simulink model "pv_mpp"  (R2023b)
settings: Solver=ode23tb  StartTime=0.0  StopTime=inf  FixedStep=0.001  MaxStep=1e-4  RelTol=1e-4
libraries: spsSeriesRLCBranchLib x4, spsCurrentMeasurementLib x1, spsDiodeLib x1, spsIGBTDiodeLib x1, spsPVArrayLib x1, spsPWMGeneratorDCDCLib x1, spsVoltageMeasurementLib x1, sps_lib x1
settings Model: Creator=SAUMYA  LastModifiedBy=SAUMYA

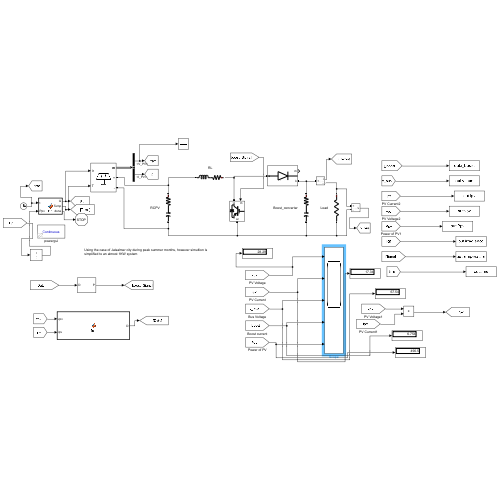
[thumbnail: Simulink's stored preview of the top-level diagram]
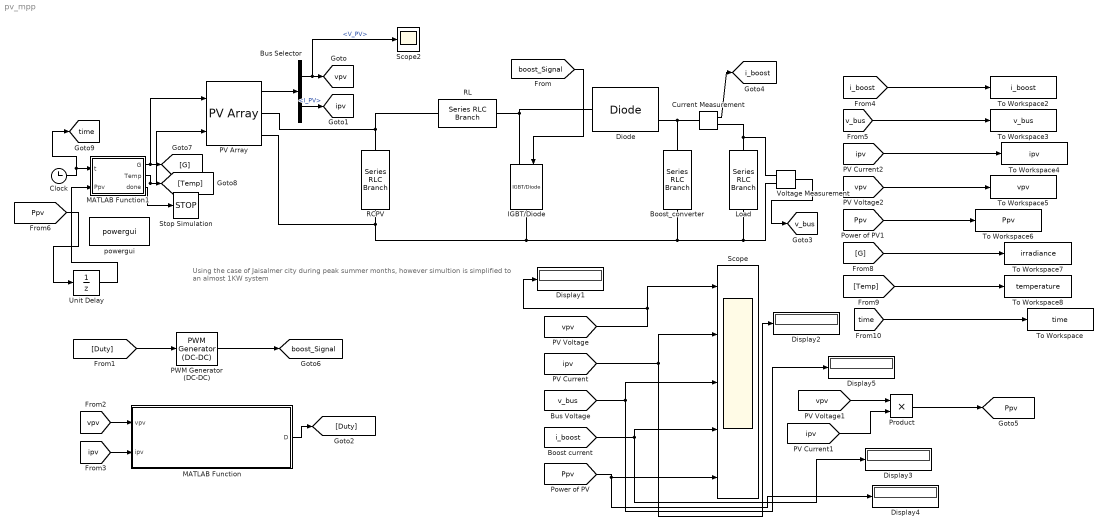
== system pv_mpp ==
  note: Using the case of Jaisalmer city during peak summer months, however simultion is simplified to an almost 1KW system
  Boost_converter : spsSeriesRLCBranchLib/Series RLC Branch  LConnTagsString=__new0  RConnTagsString=__new0  BranchType=RC  Resistance=1e-4  Inductance=1e-3  SetiL0=off  InitialCurrent=0  Capacitance=3300e-6  Setx0=on  InitialVoltage=0  Measurements=None
  Bus Selector : BusSelector  OutputSignals=V_PV,I_PV
  Clock : Clock
  Current Measurement : spsCurrentMeasurementLib/Current Measurement  PhasorSimulation=off  OutputType=Complex  PSBequivalent=0
  Diode : spsDiodeLib/Diode  Ron=0.001  Lon=0  Vf=0.8  IC=0  UseSnubber=0  Rs=inf  Cs=250e-9  Measurements=on
  Display{1..5} (5 alike) : Display
  IGBT/Diode : spsIGBTDiodeLib/IGBT//Diode  Ron=1e-3  Rs=1e5  Cs=inf  Measurements=off
  Load : spsSeriesRLCBranchLib/Series RLC Branch  LConnTagsString=__new0  RConnTagsString=__new0  BranchType=R  Resistance=10  Inductance=1e-3  SetiL0=off  InitialCurrent=0  Capacitance=3300e-6  Setx0=on  InitialVoltage=0  Measurements=None
  MATLAB Function : MATLAB Function  TreatAsAtomicUnit=on
  MATLAB Function1 : MATLAB Function  TreatAsAtomicUnit=on
  PV Array : spsPVArrayLib/PV Array  Npar=5  Nser=1  PlotType=array @ 1000 W/m2 & specified temperatures  S_vec="[ 1000  500  100 ]"  Temp_C_vec=[ 15 25 35 45 55 ]  ModuleName=Changzhou Almaden SEBP60S-220  PlotWhenSelected=off  Pm=219.876  Ncell=60  Voc=36.06  Isc=7.95  Vm=30.12  Im=7.3  beta_Voc_pc=-0.3624  alpha_Isc_pc=0.054805  beta_Voc=-0.13068  alpha_Isc=0.004357  IL=7.9642  I0=2.8692e-10  nI=0.97455  Rsh=106.1817  Rs=0.18964  RobustModel=off  RobustCellTemperature=313.3991  BAL=on  Tc=1e-6  Tfilter=5e-5
  PWM Generator (DC-DC) : spsPWMGeneratorDCDCLib/PWM Generator (DC-DC)  Fsw=5000  Ts=10e-6
  Product : Product
  RCPV : spsSeriesRLCBranchLib/Series RLC Branch  LConnTagsString=__new0  RConnTagsString=__new0  BranchType=RC  Resistance=1e-4  Inductance=1e-3  SetiL0=off  InitialCurrent=0  Capacitance=100e-6  Setx0=on  InitialVoltage=0  Measurements=None
  RL : spsSeriesRLCBranchLib/Series RLC Branch  LConnTagsString=__new0  RConnTagsString=__new0  BranchType=RL  Resistance=0.1  Inductance=5e-3  SetiL0=off  InitialCurrent=0  Capacitance=1e-3  Setx0=on  InitialVoltage=0  Measurements=None
  Scope : Scope  NumInputPorts=5
  Scope2 : Scope
  Stop Simulation : Stop
  To Workspace : ToWorkspace  VariableName=time  SampleTime=-1
  To Workspace2 : ToWorkspace  VariableName=i_boost  SampleTime=-1
  To Workspace3 : ToWorkspace  VariableName=v_bus  SampleTime=-1
  To Workspace4 : ToWorkspace  VariableName=ipv  SampleTime=-1
  To Workspace5 : ToWorkspace  VariableName=vpv  SampleTime=-1
  To Workspace6 : ToWorkspace  VariableName=Ppv  SampleTime=-1
  To Workspace7 : ToWorkspace  VariableName=irradiance  SampleTime=-1
  To Workspace8 : ToWorkspace  VariableName=temperature  SampleTime=-1
  Unit Delay : UnitDelay  SampleTime=-1  HasFrameUpgradeWarning=on
  Voltage Measurement : spsVoltageMeasurementLib/Voltage Measurement  PhasorSimulation=off  OutputType=Complex  PSBequivalent=0
  powergui : sps_lib/powergui  Priority=1  SimulationMode=Continuous  SampleTime=0.001  frequency=60  Iterations=50  frequencyindice=0  Pbase=100e6  ErrMax=1e-4  UnitsV=kV  UnitsW=MW  buscounter=0  FunctionMessages=off  echomessages=off  EnableUseOfTLC=off  CurrentSourceSwitches=off  DisableSnubberDevices=off  DisableRonSwitches=off  DisableVfSwitches=off  DisplayEquations=off  AutomaticDiscreteSolvers=off  SolverType=Tustin/Backward Euler (TBE)  Interpol=off  ExternalGateDelay=off  methode=off  Ts=100  x0status=blocks  SPID=on  SwTol=0  HookPort=off  NonlinearTolerance=1e-4  nMaxIteration=100  ContinueOnMaxIteration=off  RestoreLinks=warning  ResistiveCurrentMeasurement=off  Frange=[0:2:500]  Ylog=off  Xlog=on  ShowGrid=off  save=off  variable=ZData  structure=0  ZoomFFT=off  StartTime=0.0  cycles=1  DisplayStyle=1  fundamental=60  FreqAxis=off  MaxFrequency=1000  frequencyindicesteady=1  RmsSteady=1  display=off
  tag scope: Ppv=global, boost_Signal=global, i_boost=global, ipv=global, time=global, v_bus=global, vpv=global
  wires:
  Clock/1 -> [time], MATLAB Function1/1(t)
  MATLAB Function1/1(G) -> PV Array/1, [G]
  PWM Generator (DC-DC)/1 -> [boost_Signal]
  Current Measurement/1 -> [i_boost]
  [ipv] -> MATLAB Function/2(ipv)
  [vpv] -> Display1/1, Scope/1
  MATLAB Function1/2(Temp) -> PV Array/2, [Temp]
  [ipv] -> Product/2
  Bus Selector/1 -> Scope2/1, [vpv]  "<V_PV>"
  [v_bus] -> Display5/1, Scope/3
  [Duty] -> PWM Generator (DC-DC)/1
  Product/1 -> [Ppv]
  [boost_Signal] -> IGBT/Diode/1
  [i_boost] -> Display3/1, Scope/4
  [Ppv] -> Display4/1, Scope/5
  PV Array/1 -> Bus Selector/1
  MATLAB Function/1(D) -> [Duty]
  [vpv] -> MATLAB Function/1(vpv)
  [ipv] -> Display2/1, Scope/2
  [vpv] -> Product/1
  Voltage Measurement/1 -> [v_bus]
  Bus Selector/2 -> [ipv]  "<I_PV>"
  [i_boost] -> To Workspace2/1
  [v_bus] -> To Workspace3/1
  [ipv] -> To Workspace4/1
  [vpv] -> To Workspace5/1
  [Ppv] -> To Workspace6/1
  [G] -> To Workspace7/1
  [Temp] -> To Workspace8/1
  [time] -> To Workspace/1
  [Ppv] -> Unit Delay/1
  Unit Delay/1 -> MATLAB Function1/2(Ppv)
  MATLAB Function1/3(done) -> Stop Simulation/1
  connections:
  RCPV/LConn1 -- RL/RConn1 -- PV Array/RConn1
  RCPV/RConn1 -- Boost_converter/RConn1 -- Load/RConn1 -- Voltage Measurement/LConn2 -- IGBT/Diode/RConn1 -- PV Array/RConn2
  Current Measurement/LConn1 -- Diode/RConn1 -- Boost_converter/LConn1
  IGBT/Diode/LConn1 -- Diode/LConn1 -- RL/LConn1
  Load/LConn1 -- Voltage Measurement/LConn1 -- Current Measurement/RConn1

== matlab function pv_mpp/MATLAB Function1 ==
  settings: updateMethod=DISCRETE  sampleTime=1e-4
  data: t input; G output; Temp output; Ppv input; done output
function [G, Temp, done] = fcn(t,Ppv)
%#codegen
[G, Temp, done] = GenerateInputs(t, Ppv);
end

== matlab function pv_mpp/MATLAB Function ==
  settings: updateMethod=DISCRETE
  data: D output; vpv input; ipv input
function D  = fcn(vpv,ipv)
%#codegen

[D] = po_mppt(vpv,ipv);
end
